simulink model "matfunc"  (R2021a)
settings: Solver=VariableStepAuto  StartTime=0.0  StopTime=10.0  RelTol=1e-3
settings Model: Creator=Araz  LastModifiedBy=Araz

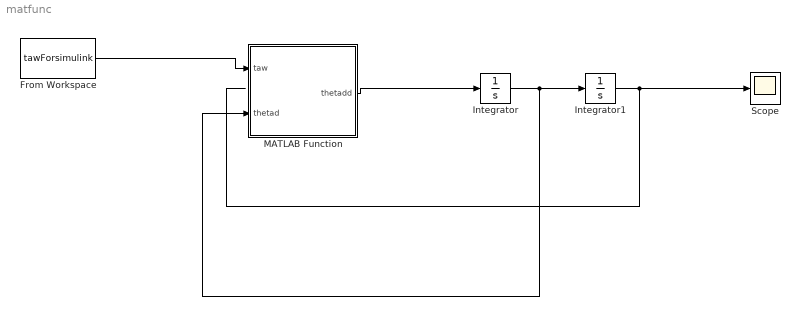
== system matfunc ==
  From Workspace : FromWorkspace  VariableName=tawForsimulink
  Integrator : Integrator
  Integrator1 : Integrator
  MATLAB Function : MATLAB Function  TreatAsAtomicUnit=on
  Scope : Scope
  wires:
  MATLAB Function/1(thetadd) -> Integrator/1
  Integrator/1 -> MATLAB Function/2(thetad), Integrator1/1
  Integrator1/1 -> Scope/1
  From Workspace/1 -> MATLAB Function/1(taw)

== matlab function matfunc/MATLAB Function ==
  data: taw input; thetadd output; thetad input
function thetadd = fcn(taw,thetad)


thetadd=(taw- C*thetad - G)/M;
